simulink model "lookupnddirect_test"  (Simulink 8.7)
settings: Solver=ode45  StartTime=0.0  StopTime=10.0  RelTol=1e-3
settings Model: Creator=arnaud  LastModifiedBy=hamza
settings DataIOCC: SaveFormat=Structure  SignalLoggingSaveFormat=ModelDataLogs
settings OptimizationCC: ExpressionDepthLimit=2147483647
settings DebuggingCC: SolverPrmCheckMsg=warning  FcnCallInpInsideContextMsg=UseLocalSettings  StateNameClashWarn=warning
settings GRTTargetCC: CombineOutputUpdateFcns=off  GRTInterface=on
settings ConfigComp: CovSFcnEnable=off

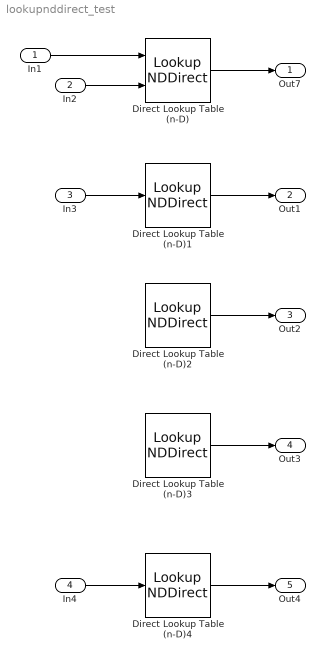
== system lookupnddirect_test ==
  In1 : Inport  OutDataTypeStr=int8  PortDimensions=1
  In2 : Inport  Port=2  OutDataTypeStr=int8  PortDimensions=1
  In3 : Inport  Port=3  OutDataTypeStr=int8  PortDimensions=1
  In4 : Inport  Port=4  OutDataTypeStr=int8  PortDimensions=1
  Direct Lookup Table (n-D) : LookupNDDirect
  Direct Lookup Table (n-D)1 : LookupNDDirect  NumberOfTableDimensions=1  Table=[4 5 6]
  Direct Lookup Table (n-D)2 : LookupNDDirect  NumberOfTableDimensions=1  InputsSelectThisObjectFromTable=Column  Table=[4 5 6]
  Direct Lookup Table (n-D)3 : LookupNDDirect  InputsSelectThisObjectFromTable=2-D Matrix  Table=[4 5 6; 7 8 9]
  Direct Lookup Table (n-D)4 : LookupNDDirect  InputsSelectThisObjectFromTable=Column  Table=[4 5 6; 7 8 9]
  Out7 : Outport
  Out1 : Outport  Port=2
  Out2 : Outport  Port=3
  Out3 : Outport  Port=4
  Out4 : Outport  Port=5
  wires:
  In1/1 -> Direct Lookup Table (n-D)/1
  In2/1 -> Direct Lookup Table (n-D)/2
  Direct Lookup Table (n-D)/1 -> Out7/1
  In3/1 -> Direct Lookup Table (n-D)1/1
  Direct Lookup Table (n-D)1/1 -> Out1/1
  Direct Lookup Table (n-D)2/1 -> Out2/1
  Direct Lookup Table (n-D)3/1 -> Out3/1
  Direct Lookup Table (n-D)4/1 -> Out4/1
  In4/1 -> Direct Lookup Table (n-D)4/1
